simulink model "snap_fengine"  (R2016b)
settings: Solver=VariableStepDiscrete  StartTime=0.0  StopTime=10.0  RelTol=1e-3
libraries: xbsIndex_r4 x5026, casper_library_misc x38, xps_library x10, casper_library_delays x6, casper_library_sources x3, casper_library_reorder x2, casper_library_communications x1
(part 1 of 43)
settings Model: Creator=mdexter  LastModifiedBy=jackh
settings Model: ModifiedComment=|
  | jackh -- Sun Oct 27 09:17:26 2019 -- Version 1.368
  | compiled
settings Model: ModifiedHistory=|
  | jackh -- Sun Oct 27 09:17:26 2019 -- Version 1.368
  | compiled
  | 
  | jackh -- Sun Oct 27 07:24:12 2019 -- Version 1.367
  | remove registering of reorder outputs
  | 
  | jackh -- Sun Oct 27 07:22:37 2019 -- Version 1.366
  | change input snapshot to snap only one of 3 inputs
  | 
  | jackh -- Sun Oct 27 03:59:18 2019 -- Version 1.365
  | remove some superfluous registers to improve timing.
  | Reduce snapshot in input block from 1k samples to 512
  | 
  | jackh -- Sun Oct 27 01:46:50 2019 -- Version 1.364
  | Fix FFT shift bitwidth bug
  | 
  | FFT core was expecting a 16-bit shift, but only a 12bit value was sliced from the control register
  | 
  | jackh -- Fri Aug 30 09:22:01 2019 -- Version 1.363
  | compiled
  | 
  | jackh -- Thu Aug 29 17:13:27 2019 -- Version 1.362
  | change delay shift reg to 3 bit addr
  | 
  | jackh -- Thu Aug 29 11:33:13 2019 -- Version 1.361
  | corr fixes
  | 
  | jackh -- Thu Aug 29 11:09:21 2019 -- Version 1.360
  | latency fix in eqtvg
  | 
  | jackh -- Thu Aug 29 10:02:04 2019 -- Version 1.359
  | compiled
  | 
  | jackh -- Wed Aug 28 15:31:00 2019 -- Version 1.358
  | bump to version 1.3
  | 
  | jackh -- Wed Aug 28 15:26:18 2019 -- Version 1.357
  | change quantization to saturate.
  | Change coefficients to 16_5 (was 16_6)
  | 
  | jackh -- Wed Aug 28 14:17:28 2019 -- Version 1.356
  | remove debugging snapshots hidden in corr vaccs
  | 
  | jackh -- Fri Aug 23 15:01:55 2019 -- Version 1.355
  | compiled
  | 
  | jackh -- Fri Aug 23 10:43:05 2019 -- Version 1.354
  | add snapshot in input block
  | 
  | jackh -- Thu Aug 22 17:13:50 2019 -- Version 1.353
  | fix to eqtvg ram depths
  | 
  | jackh -- Thu Aug 22 15:23:14 2019 -- Version 1.352
  | bump version to 1.2
  | 
  | jackh -- Thu Aug 22 15:22:39 2019 -- Version 1.351
  | Force pairs of pols to have same random number generator to save resources
  | 
  | jackh -- Thu Aug 22 15:19:21 2019 -- Version 1.350
  | rotator channel index counter fixes
  | 
  | eq tvg split bram into 3 (so we can have 6 channels, not 8)
  | 
  | jackh -- Thu Aug 22 12:01:44 2019 -- Version 1.349
  | 
  | 
  | jackh -- Thu Aug 22 12:01:21 2019 -- Version 1.348
  | Changes to rotator precision
  | 
  | jackh -- Tue Aug 20 19:46:09 2019 -- Version 1.347
  | compiled
  | 
  | jackh -- Tue Aug 20 16:55:38 2019 -- Version 1.346
  | increase minimum walsh period to 2**18 fpga clocks (was 2**13)
  | 
  | jackh -- Tue Aug 20 16:40:34 2019 -- Version 1.345
  | 
  | 
  | jackh -- Tue Aug 20 16:15:18 2019 -- Version 1.344
  | bump version to 1.1
  | 
  | jackh -- Tue Aug 20 16:14:49 2019 -- Version 1.343
  | add global enables to phase switch mod/demod to make software easier
  | 
  | jackh -- Mon Aug 19 17:54:23 2019 -- Version 1.342
  | compiled
  | 
  | jackh -- Thu Aug 01 11:53:22 2019 -- Version 1.341
  | make programmable sync delay tolerate delay=0
  | 
  | jackh -- Wed Jul 31 13:49:54 2019 -- Version 1.340
  | comment out corr->rms
  | 
  | jackh -- Mon Jul 29 17:05:34 2019 -- Version 1.339
  | delete corr rms block (not currently enough ram)
  | 
  | jackh -- Mon Jul 29 17:03:29 2019 -- Version 1.338
  | Add version block
  | 
  | jackh -- Mon Jul 29 16:58:22 2019 -- Version 1.337
  | make sync in have a programmable delay
  | Solves 2 problems:
  | 
  | 1) Can start integrations at arbitrary times (good for LST alignment)
  | 2) Can start a 16 second integration chunk on an arbitrary time boundary (needed to avoid the downstream correlator having 16 second start / stop granularity)
  | 
  | jackh -- Mon Jul 29 16:50:03 2019 -- Version 1.336
  | update phasor to 24-bits
  | 
  | jackh -- Sat May 11 17:48:41 2019 -- Version 1.335
  | 
  | 
  | jackh -- Sat May 11 17:46:07 2019 -- Version 1.334
  | 
  | 
  | jackh -- Sat May 11 17:45:44 2019 -- Version 1.333
  | 
  | 
  | jackh -- Sat May 11 17:40:04 2019 -- Version 1.332
  | 
  | 
  | jackh -- Sat May 11 17:36:59 2019 -- Version 1.331
  | add vacc for autocorrs @ 16 bit resolution
  | 
  | deepthi -- Sun Oct 28 15:16:19 2018 -- Version 1.330
  | 
  | 
  | deepthi -- Sat Oct 27 18:45:54 2018 -- Version 1.329
  | 
  | packetizer: Added an 'and' block that holds new_packet signal in high until the first sync.
  | 
  | deepthi -- Sat Oct 27 17:33:32 2018 -- Version 1.328
  | 
  | 1. Change edge_detect location in sync block
  | 
  | deepthi -- Sat Oct 20 22:13:43 2018 -- Version 1.327
  | 
  | 1. Add edge detect to software reg and gpio input in sync block.
  | 
  | 2. Add new corr block with max hold functionality.
  | 
  | jackh -- Tue Oct 09 20:34:13 2018 -- Version 1.326
  | recompile with pmbus_alert register
  | 
  | jackh -- Thu Jul 12 10:55:28 2018 -- Version 1.325
  | 
  | 
  | jackh -- Wed Jul 11 17:20:51 2018 -- Version 1.324
  | syntax
  | 
  | jackh -- Wed Jul 11 17:16:24 2018 -- Version 1.323
  | increase resolution of phase rotator bram.
  | 
  | jackh -- Wed Jul 11 17:10:41 2018 -- Version 1.322
  | 
  | 
  | jackh -- Tue Jul 10 16:08:30 2018 -- Version 1.321
  | scramble rotator channel multiplers to match PFB output order (hopefully)
  | 
  | jackh -- Tue Jul 10 15:51:56 2018 -- Version 1.320
  | 
  | 
  | jackh -- Tue Jul 10 13:37:24 2018 -- Version 1.319
  | fix off-by-one in slicing of mcnt counter, which was having the effect of duplicating mcnts in headers
  | 
  | jackh -- Sat Jul 07 14:17:05 2018 -- Version 1.318
  | compiled
  | 
  | jackh -- Fri Jul 06 10:33:47 2018 -- Version 1.317
  | fix bitbashing to rotator phase addresses
  | 
  | jackh -- Fri Jul 06 10:17:15 2018 -- Version 1.316
  | Add mux to enable / disable rotator
  | 
  | jackh -- Thu Jul 05 17:21:10 2018 -- Version 1.315
  | make some delays behavioural
  | 
  | jackh -- Thu Jul 05 14:48:28 2018 -- Version 1.314
  | 
  | 
  | jackh -- Thu Jul 05 14:46:13 2018 -- Version 1.313
  | 
  | 
  | jackh -- Thu Jul 05 14:43:36 2018 -- Version 1.312
  | 
  | 
  | jackh -- Thu Jul 05 14:40:00 2018 -- Version 1.311
  | 
  | 
  | jackh -- Thu Jul 05 14:36:19 2018 -- Version 1.310
  | 
  | 
  | jackh -- Thu Jul 05 14:26:16 2018 -- Version 1.309
  | integrate rotator into pipeline
  | 
  | jackh -- Thu Jul 05 14:20:20 2018 -- Version 1.308
  | 
  | create phase-rotation block
  | 
  | deepthi -- Thu Jun 07 09:24:03 2018 -- Version 1.307
  | 
  | Replaced the corr block.
  | 
  | deepthi -- Wed Jun 06 12:07:26 2018 -- Version 1.306
  | 
  | 
  | deepthi -- Tue Jun 05 17:46:17 2018 -- Version 1.305
  | 
  | Replaced the corr block with the tested version
  | 
  | deepthi -- Sat May 12 19:11:02 2018 -- Version 1.304
  | 
  | Changed time counter to increment between even/odd banks
  | 
  | deepthi -- Sat May 12 19:06:34 2018 -- Version 1.303
  | 
  | changed timing of eof, valid, data and headers
  | 
  | deepthi -- Mon May 07 23:03:07 2018 -- Version 1.302
  | 
  | 
  | deepthi -- Mon May 07 00:31:44 2018 -- Version 1.301
  | 
  | 
  | deepthi -- Fri May 04 20:13:43 2018 -- Version 1.300
  | 
  | Reduced width sliced from time_ctr
  | 
  | deepthi -- Fri May 04 19:47:57 2018 -- Version 1.299
  | 
  | Added delay to header and ip signals to account for pulse_ext on valid.
  | 
  | deepthi -- Fri May 04 19:23:23 2018 -- Version 1.298
  | 
  | 
  | deepthi -- Thu May 03 16:58:39 2018 -- Version 1.297
  | 
  | 1. Added delays to eof and dest_ip  to account for pulse_ext in valid.
  | 
  | 2. Changed eth_sw expected packet length to include header.
  | 
  | jackh -- Tue May 01 20:38:09 2018 -- Version 1.296
  | compiled
  | 
  | jackh -- Tue May 01 17:49:38 2018 -- Version 1.295
  | Fix to packetizer valid generation, to take into account the 3 (one per antenna) blocks of valid data in each stream of 512 channels
  | 
  | jackh -- Tue May 01 16:49:02 2018 -- Version 1.294
  | make channel selection bram 32-bits wide.
  | 
  | Remove GPU-packing mux / swreg
  | 
  | jackh -- Tue May 01 14:24:16 2018 -- Version 1.293
  | 
  | 
  | jackh -- Tue May 01 14:20:01 2018 -- Version 1.292
  | update chan reorderer
  | 
  | jackh -- Tue May 01 11:43:41 2018 -- Version 1.291
  | compiled
  | 
  | jackh -- Tue May 01 09:44:03 2018 -- Version 1.290
  | 
  | 
  | jackh -- Tue May 01 09:43:34 2018 -- Version 1.289
  | use bram for eq fft descramble map
  | 
  | jackh -- Tue May 01 09:40:26 2018 -- Version 1.288
  | change architecture of corr block -- now stores desired antennas in bram, rather than using a delay tree
  | 
  | jackh -- Mon Apr 30 20:21:35 2018 -- Version 1.287
  | 
  | 
  | jackh -- Mon Apr 30 20:18:20 2018 -- Version 1.286
  | 
  | 
  | jackh -- Mon Apr 30 20:15:51 2018 -- Version 1.285
  | compensate for FFT scrambling in EQ block. Descramble FFT post-requantization in this block
  | 
  | jackh -- Mon Apr 30 19:27:42 2018 -- Version 1.284
  | plausibility pass on corr block
  | 
  | jackh -- Mon Apr 30 12:16:47 2018 -- Version 1.283
  | 
  | 
  | jackh -- Mon Apr 30 12:14:25 2018 -- Version 1.282
  | store chan_reorder reorder map in bram
  | 
  | jackh -- Mon Apr 30 12:05:02 2018 -- Version 1.281
  | remove per-antenna histograms -- now get one histogram with multiplexed input
  | 
  | jackh -- Sun Apr 29 15:50:16 2018 -- Version 1.280
  | 
  | 
  | jackh -- Sun Apr 29 15:37:38 2018 -- Version 1.279
  | 
  | 
  | jackh -- Sun Apr 29 15:27:38 2018 -- Version 1.278
  | First pass packetizer. Regenerate pfb with parameter for serial block inputs
  | 
  | jackh -- Sat Mar 03 12:52:57 2018 -- Version 1.277
  | 
  | 
  | jackh -- Sun Feb 25 12:27:48 2018 -- Version 1.276
  | add pre-pfb reorder
  | 
  | jackh -- Sat Feb 24 13:39:06 2018 -- Version 1.275
  | 
  | jackh -- Sat Feb 24 13:38:40 2018 -- Version 1.274
  | update pfb to 16 inputs
  | 
  | jackh -- Fri Feb 23 18:44:26 2018 -- Version 1.273
  | 
  | 
  | jackh -- Fri Feb 23 18:38:20 2018 -- Version 1.272
  | 
  | 
  | jackh -- Fri Feb 23 17:01:30 2018 -- Version 1.271
  | make fft 8 parallel input
  | 
  | jackh -- Sat Feb 10 13:53:12 2018 -- Version 1.270
  | 
  | 
  | jackh -- Sat Feb 10 13:50:10 2018 -- Version 1.269
  | 
  | 
  | jackh -- Sat Feb 10 13:48:56 2018 -- Version 1.268
  | remove fft preshift
  | 
  | jackh -- Sat Feb 10 13:47:39 2018 -- Version 1.267
  | 
  | 
  | jackh -- Sat Feb 10 13:44:29 2018 -- Version 1.266
  | 
  | 
  | jackh -- Sat Feb 10 13:43:22 2018 -- Version 1.265
  | make delayer dual-pol
  | 
  | jackh -- Sat Feb 10 13:40:59 2018 -- Version 1.264
  | first pass new packet format with no time-based corner turn
  | 
  | jackh -- Fri Feb 09 17:29:05 2018 -- Version 1.263
  | 
  | 
  | jackh -- Fri Feb 09 15:23:03 2018 -- Version 1.262
  | first pass turning everything to 8192 channels
  | 
  | Changed the ants addr to be driven by the same signal that drives chans, ips (used to be driven by ant_tracker).
  | 
  | Removed nants software register that was previously thought to control time stamps (but didn't really)
  | 
  | deepthi -- Wed Jan 31 18:20:45 2018 -- Version 1.261
  | 
  | deepthi -- Mon Jan 29 17:20:36 2018 -- Version 1.260
  | 
  | 
  | deepthi -- Mon Jan 29 17:18:54 2018 -- Version 1.259
  | 
  | 
  | deepthi -- Mon Jan 29 17:18:33 2018 -- Version 1.258
  | 
  | 
  | deepthi -- Mon Jan 29 16:51:19 2018 -- Version 1.257
  | 
  | 
  | deepthi -- Mon Jan 29 16:46:46 2018 -- Version 1.256
  | 
  | 
  | deepthi -- Mon Jan 29 16:37:32 2018 -- Version 1.255
  | 
  | 
  | deepthi -- Mon Jan 29 16:11:03 2018 -- Version 1.254
  | 
  | 
  | deepthi -- Mon Jan 29 15:55:33 2018 -- Version 1.253
  | 
  | 
  | jackh -- Fri Nov 17 19:04:05 2017 -- Version 1.252
  | compiled
  | 
  | jackh -- Wed Nov 15 11:31:03 2017 -- Version 1.251
  | go to 3 corr blocks
  | 
  | jackh -- Tue Nov 14 16:10:40 2017 -- Version 1.250
  | 
  | 
  | jackh -- Tue Nov 14 15:28:37 2017 -- Version 1.249
  | reduce bram use in histogram shared brams
  | 
  | jackh -- Mon Nov 13 18:55:18 2017 -- Version 1.248
  | fix bug in histogram shared bram addr width
  | 
  | jackh -- Fri Nov 10 17:05:56 2017 -- Version 1.247
  | add 4 independent corr subsystems. Add EQ clipping counters
  | 
  | jackh -- Fri Nov 10 14:21:14 2017 -- Version 1.246
  | 
  | 
  | jackh -- Fri Nov 10 14:19:27 2017 -- Version 1.245
  | 
  | 
  | jackh -- Fri Nov 10 11:40:47 2017 -- Version 1.244
  | update to histograms v2
  | 
  | jackh -- Tue Nov 07 22:23:59 2017 -- Version 1.243
  | compiled -- passes eqtvg
  | 
  | jackh -- Tue Nov 07 20:41:00 2017 -- Version 1.242
  | 
  | 
  | jackh -- Tue Nov 07 20:39:30 2017 -- Version 1.241
  | packet header generation fixes
  | 
  | jackh -- Tue Nov 07 17:19:53 2017 -- Version 1.240
  | 
  | 
  | jackh -- Tue Nov 07 17:14:47 2017 -- Version 1.239
  | 
  | 
  | jackh -- Tue Nov 07 17:08:29 2017 -- Version 1.238
  | remove some chan_reorder debug snapshots
  | 
  | jackh -- Tue Nov 07 17:06:39 2017 -- Version 1.237
  | update ps GPIO pins
  | 
  | **** Change packetizer header blocks to can have a separate antenna / ip / chan for each packet. This is for the nants > 3 simulation modes. This will break previous versions of software *****
  | 
  | jackh -- Mon Nov 06 22:06:03 2017 -- Version 1.236
  | add comment to corr_acc_len
  | 
  | Compiled -- passes EQTVG test!
  | 
  | jackh -- Mon Nov 06 15:24:31 2017 -- Version 1.235
  | add OR block in mrst generator so that counter is enabled if/when an arm signal comes
  | 
  | jackh -- Sun Nov 05 21:39:25 2017 -- Version 1.234
  | comment on sync period
  | 
  | jackh -- Sun Nov 05 17:39:01 2017 -- Version 1.233
  | fix bitbasher in 32-spectra corner turn
  | 
  | jackh -- Sun Nov 05 17:05:17 2017 -- Version 1.232
  | aesthetic
  | 
  | jackh -- Sun Nov 05 17:02:53 2017 -- Version 1.231
  | changes to comments
  | 
  | jackh -- Sun Nov 05 17:01:27 2017 -- Version 1.230
  | make acc_len it's own register so we can acc to 2**32
  | 
  | jackh -- Sun Nov 05 16:58:57 2017 -- Version 1.229
  | 
  | 
  | jackh -- Sun Nov 05 16:56:52 2017 -- Version 1.228
  | add internal correlator
  | 
  | jackh -- Sun Nov 05 16:24:21 2017 -- Version 1.227
  | compiled.
  | 
  | jackh -- Sun Nov 05 15:19:13 2017 -- Version 1.226
  | latency tweak to data line in packetizer
  | 
  | jackh -- Sat Nov 04 20:21:54 2017 -- Version 1.225
  | change ethernet debug counters to 32 bits
  | 
  | jackh -- Sat Nov 04 20:05:10 2017 -- Version 1.224
  | make chan reorder map bram 32 bits to aid with software
  | 
  | jackh -- Sat Nov 04 19:51:25 2017 -- Version 1.223
  | change header brams to be 32-bit wide for all values.
  | This makes it easier to deal with the software, which can only write 32-bit bounded words.
  | 
  | jackh -- Sat Nov 04 14:23:39 2017 -- Version 1.222
  | replace big distributed ram in 16-spectra corner turn
  | with simple bit basher manipulation. The distributed ram tool a ridiculous amount of time to synthesize. Hopefully this will be faster.
  | 
  | jackh -- Fri Nov 03 16:25:40 2017 -- Version 1.221
  | 
  | 
  | jackh -- Fri Nov 03 16:17:13 2017 -- Version 1.220
  | update casper blocks on phase switch subsys
  | 
  | jackh -- Fri Nov 03 16:14:34 2017 -- Version 1.219
  | 
  | 
  | jackh -- Fri Nov 03 13:09:23 2017 -- Version 1.218
  | add phase switching and i2c control
  | 
  | jackh -- Fri Nov 03 12:43:29 2017 -- Version 1.217
  | 
  | add i2C controllers
  | 
  | jackh -- Mon Oct 23 16:15:14 2017 -- Version 1.216
  | Add back in Deepthi's fix from f3b63dae07d62
  | 
  | jackh -- Mon Oct 23 16:04:59 2017 -- Version 1.215
  | 
  | 
  | jackh -- Mon Oct 23 14:44:02 2017 -- Version 1.214
  | compiled. Still minor timing errors in the histograms
  | 
  | jackh -- Mon Oct 23 10:40:37 2017 -- Version 1.213
  | change EQ coeffs to one-per channel. Make format 16_6 (was 18_7)
  | 
  | jackh -- Mon Oct 09 15:00:17 2017 -- Version 1.212
  | 
  | halve number of brams in histogram readout
  | 
  | jackh -- Wed Sep 13 11:46:17 2017 -- Version 1.211
  | use built-in tge status regs
  | 
  | jackh -- Tue Sep 12 21:14:25 2017 -- Version 1.210
  | 
  | 
  | jackh -- Tue Sep 12 21:10:57 2017 -- Version 1.209
  | update_casper_blocks(bdroot)
  | 
  | jackh -- Tue Sep 12 21:02:11 2017 -- Version 1.208
  | add histogram to adc stats
  | 
  | jackh -- Fri Jul 14 11:30:38 2017 -- Version 1.207
  | set map = reord_map in chan_reorder blocks which use matlab scripts to generate their reorders.
  | 
  | jackh -- Thu Jul 13 17:48:05 2017 -- Version 1.206
  | change sync period to a 32-bit sw reg (was hardcoded 9! * 1024)
  | 
  | deepthi -- Thu Jul 13 13:07:36 2017 -- Version 1.205
  | 
  | 
  | deepthi -- Thu Jul 13 12:10:35 2017 -- Version 1.204
  | 
  | 
  | deepthi -- Wed Jul 12 16:52:46 2017 -- Version 1.203
  | 
  | 
  | deepthi -- Wed Jul 12 15:57:48 2017 -- Version 1.202
  | 
  | 
  | deepthi -- Tue Jul 11 19:00:41 2017 -- Version 1.201
  | 
  | 
  | deepthi -- Tue Jul 11 18:54:05 2017 -- Version 1.200
  | 
  | 
  | deepthi -- Tue Jul 11 18:52:32 2017 -- Version 1.199
  | 
  | 
  | deepthi -- Mon Jul 10 16:18:51 2017 -- Version 1.198
  | 
  | 
  | deepthi -- Sun Jul 09 18:15:02 2017 -- Version 1.197
  | 
  | 
  | deepthi -- Thu Jul 06 13:54:16 2017 -- Version 1.196
  | 
  | 
  | jackh -- Mon Jul 03 11:01:40 2017 -- Version 1.195
  | 
  | 
  | jackh -- Fri Jun 30 13:59:17 2017 -- Version 1.194
  | enable CPU tx/rx buffer on tge core. Needed for microblaze.
  | 
  | jackh -- Mon Jun 26 11:33:24 2017 -- Version 1.193
  | 
  | 
  | jackh -- Thu Jun 22 14:37:16 2017 -- Version 1.192
  | add history prompting
settings DataIOCC: LimitDataPoints=on  SaveFormat=Array  SignalLoggingSaveFormat=ModelDataLogs
settings OptimizationCC: DefaultParameterBehavior=Inlined  ExpressionDepthLimit=2147483647  LifeSpan=inf
settings DebuggingCC: UnderspecifiedInitializationDetection=Classic  MergeDetectMultiDrivingBlocksExec=none  SolverPrmCheckMsg=warning  FcnCallInpInsideContextMsg=warning  AllowSymbolicDim=off  StateNameClashWarn=warning  SFUnexpectedBacktrackingDiag=warning  SFNoUnconditionalDefaultTransitionDiag=warning  SFExecutionAtInitializationDiag=none
settings HardwareCC: ProdBitPerPointer=32  ProdBitPerSizeT=32  ProdBitPerPtrDiffT=32  ProdLargestAtomicFloat=None  ProdIntDivRoundTo=Undefined  ProdEndianess=Unspecified  ProdWordSize=32  ProdHWDeviceType=32-bit Generic
settings ModelReferenceCC: PropagateSignalLabelsOutOfModel=off
settings GRTTargetCC: TargetLangStandard=C89/C90 (ANSI)  GeneratePreprocessorConditionals=Disable all  CombineOutputUpdateFcns=off  GRTInterface=on
settings ConfigComp: CovMetricSettings=dw  CovHtmlReporting=on  CovSaveCumulativeToWorkspaceVar=on  CovSaveSingleToWorkspaceVar=on  CovExternalEMLEnable=off

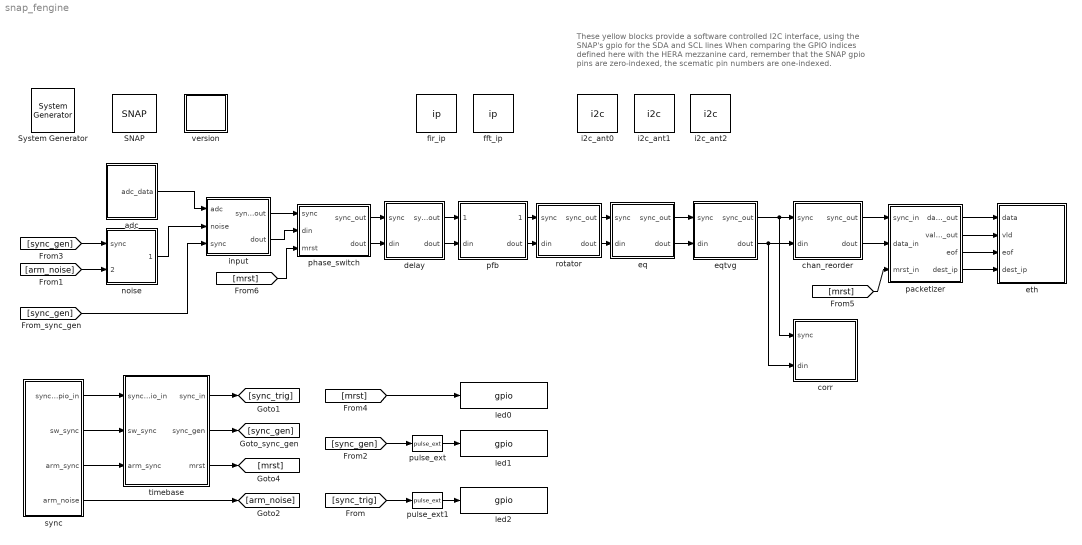
== system snap_fengine ==
  note: These yellow blocks provide a software controlled I2C interface, using
      | the SNAP's gpio for the SDA and SCL lines
      | When comparing the GPIO indices defined here with the HERA
      | mezzanine card, remember that the SNAP gpio pins are zero-indexed,
      | the scematic pin numbers are one-indexed.
  " System Generator" : xbsIndex_r4/ System Generator  Tag=genX  xilinxfamily=kintex7  part=xc7k160t  speed=-2  package=ffg676  synthesis_tool=XST  clock_wrapper=Clock Enables  directory=/data/home/jackh/herafengine/snap_fengine/sysgen  proj_type=Vivado  Synth_file=Vivado Synthesis Defaults  Impl_file=Vivado Implementation Defaults  testbench=off  simulink_period=1  sysclk_period=4  dcm_input_clock_period=10  incr_netlist=off  trim_vbits=Everywhere in SubSystem  dbl_ovrd=According to Block Masks  core_generation=According to Block Masks  run_coregen=off  deprecated_control=off  eval_field=0  block_type=sysgen
  SNAP : xps_library/Platforms/SNAP  Tag=xps:xsg  hw_sys=SNAP:xc7k160t  clk_src=adc0_clk  clk_rate=250  use_microblaze=on  sample_period=1  synthesis_tool=XST
  adc : Subsystem
  chan_reorder : Subsystem
  corr : Subsystem
  delay : Subsystem
  eq : Subsystem
  eqtvg : Subsystem
  eth : Subsystem
  fft_ip : xps_library/ip  Tag=xps:ip  lib_path=[fileparts(which(gcs)) '/fft_8192_1a_core']  ip_name='fft_8192_1a_core'
  fir_ip : xps_library/ip  Tag=xps:ip  lib_path=[fileparts(which(gcs)) '/pfb_fir_8192ch_core']  ip_name='pfb_fir_8192ch_core'
  i2c_ant0 : xps_library/i2c  Tag=xps:i2c  sda_gpio='rpi_header'  sda_gpio_index=6  scl_gpio='rpi_header'  scl_gpio_index=7
  i2c_ant1 : xps_library/i2c  Tag=xps:i2c  sda_gpio='rpi_header'  sda_gpio_index=30  scl_gpio='rpi_header'  scl_gpio_index=31
  i2c_ant2 : xps_library/i2c  Tag=xps:i2c  sda_gpio='rpi_header'  sda_gpio_index=35  scl_gpio='rpi_header'  scl_gpio_index=36
  input : Subsystem
  led0 : xps_library/gpio  Tag=xps:gpio  io_group=ROACH2:led  io_group_custom=0  io_dir=out  arith_type=Boolean  bitwidth=1  bin_pt=0  bit_index=0  sample_period=1  use_single_ended=off  use_ddr=off  reg_iob=on  reg_clk_phase=0  termination=None
  led1 : xps_library/gpio  Tag=xps:gpio  io_group=ROACH2:led  io_group_custom=0  io_dir=out  arith_type=Boolean  bitwidth=1  bin_pt=0  bit_index=1  sample_period=1  use_single_ended=off  use_ddr=off  reg_iob=on  reg_clk_phase=0  termination=None
  led2 : xps_library/gpio  Tag=xps:gpio  io_group=ROACH2:led  io_group_custom=0  io_dir=out  arith_type=Boolean  bitwidth=1  bin_pt=0  bit_index=2  sample_period=1  use_single_ended=off  use_ddr=off  reg_iob=on  reg_clk_phase=0  termination=None
  noise : Subsystem
  packetizer : Subsystem  mask{nchan_bits=13, nsamp_per_pkt=2, nchan_per_pkt=384, nant_per_pkt=3, nants=4, clks_per_pkt=512/8*4*2*2, pkts_per_cycle=16*2, chan_frac_sent=384/512}
      mask prompts: nchan_bits "Number of channels (including unsent) (2^?)"; nsamp_per_pkt "Time samples per packet"; nchan_per_pkt "Channels per packet"; nant_per_pkt "Antennas per packet"; nants "Number of antennas including dummys"; clks_per_pkt "Send packet every ? clocks"; pkts_per_cycle "Packets per cycle"; chan_frac_sent "Fraction of channels sent"
      mask init:
      | nwords = nchan_per_pkt * nsamp_per_pkt * nant_per_pkt * 2 / 8
      | 
      | % +1 for dual-pol => 2 bytes per sample
      | % -3 for 2^3 = 8 bytes per word
      | 
      | clks_to_eof = (512*nsamp_per_pkt*nant_per_pkt*2/8) -(512*nsamp_per_pkt*2)/(4*8)
      | 
      | % 512 (including channels not sent)
      | % -512/4. to account for (1-chan_frac_sent) valid=0
  pfb : Subsystem
  phase_switch : Subsystem
  pulse_ext : casper_library_misc/pulse_ext  pulse_len=2^26
  pulse_ext1 : casper_library_misc/pulse_ext  pulse_len=2^26
  rotator : Subsystem  mask{chan_bits=13, pchan_bits=3, npol_bits=3, spectra_share_bits=10, spectra_bits=19}
      mask prompts: chan_bits "Number of channels (2^?)"; pchan_bits "Parallel channels (2^?)"; npol_bits "Number of polarizations (2^?) (Sequential polarization pairs are assumed to be from the same antenna, and get the same phase)"; spectra_share_bits "Increment phase every how many spectra (2^?)"; spectra_bits "Maximum number of spectra to phase (2^?)"
  sync : Subsystem
  timebase : Subsystem
  version : Subsystem  mask{ver_maj=1, ver_min=4}
      mask prompts: ver_maj "Major version"; ver_min "Minor version"
  wires:
  adc/1(adc_data) -> input/1(adc)
  noise/1(noise) -> input/2(noise)
  sync/1(sync_gpio_in) -> timebase/1(sync_gpio_in)
  sync/2(sw_sync) -> timebase/2(sw_sync)
  sync/3(arm_sync) -> timebase/3(arm_sync)
  [arm_noise] -> noise/2(arm_ld)
  [sync_gen] -> noise/1(sync)
  timebase/2(sync_gen) -> [sync_gen]
  timebase/1(sync_in) -> [sync_trig]
  sync/4(arm_noise) -> [arm_noise]
  [sync_gen] -> input/3(sync)
  eq/1(sync_out) -> eqtvg/1(sync)
  eq/2(dout) -> eqtvg/2(din)
  eqtvg/1(sync_out) -> corr/1(sync), chan_reorder/1(sync)
  eqtvg/2(dout) -> corr/2(din), chan_reorder/2(din)
  packetizer/1(data_out) -> eth/1(data)
  packetizer/2(valid_out) -> eth/2(vld)
  packetizer/3(eof) -> eth/3(eof)
  packetizer/4(dest_ip) -> eth/4(dest_ip)
  timebase/3(mrst) -> [mrst]
  [sync_gen] -> pulse_ext/1
  [mrst] -> led0/1
  pulse_ext/1 -> led1/1
  delay/1(sync_out) -> pfb/1(sync_in)
  delay/2(dout) -> pfb/2(din)
  [sync_trig] -> pulse_ext1/1
  pulse_ext1/1 -> led2/1
  input/1(sync_out) -> phase_switch/1(sync)
  phase_switch/2(dout) -> delay/2(din)
  phase_switch/1(sync_out) -> delay/1(sync)
  input/2(dout) -> phase_switch/2(din)
  [mrst] -> phase_switch/3(mrst)
  chan_reorder/1(sync_out) -> packetizer/1(sync_in)
  chan_reorder/2(dout) -> packetizer/2(data_in)
  [mrst] -> packetizer/3(mrst_in)
  pfb/1(sync_out) -> rotator/1(sync)
  pfb/2(dout) -> rotator/2(din)
  rotator/1(sync_out) -> eq/1(sync)
  rotator/2(dout) -> eq/2(din)

== system snap_fengine/adc ==
  Assert{,1..11} (12 alike) : xbsIndex_r4/Assert  assert_type=off  type_source=Explicitly  gui_display_data_type=Fixed-point  arith_type="Signed  (2's comp)"  n_bits=16  bin_pt=14  preci_type=Single  exp_width=8  frac_width=24  assert_rate=on  rate_source=Explicitly  period=1  output_port=on  block_type=assert
  Constant{4..13,33..34} (12 alike) : Constant  Value=0
  bus_create : Subsystem  AncestorBlock=casper_library_flow_control/bus_create  mask(bus_create){inputNum=12}
      mask prompts: inputNum "Number of inputs:"
      mask init:
      | bus_create_init(gcb,...
      |     'inputNum', inputNum);
  snap_adc : Subsystem  Tag=xps:snap_adc  AncestorBlock=xps_library/ADCs/snap_adc  mask(adc_snap){sample_rate=500, snap_inputs=6, adc_resolution=8}
      mask prompts: sample_rate "Sample rate (MHz)"; snap_inputs "Number of inputs per snap"; adc_resolution "Resolution of ADC (number of bit)"
      mask help: Interface to the 3 adc chips on the SNAP board. Please see Help for instructions on parameter settings
      mask init:
      | adc_snap_init(gcb);
      mask Help:
      | This is the CASPER "yellow block" for the ADCs on the SNAP board.
      | Each ADC chip accepts four inputs.
      | 
      | Maximum sample rate f (Mega samples per second)
      | 
      | Number of inputs         3                6                12
      | Resolution 8 bits          f=1000      f=500         f=250
      | Resolution 12 bits        f=640        f=320         f=160
      | 
      | Resolution 12 bits is available when SNAP board is upgraded with HMCAD1520 ADC chips
      mask TypeOptions snap_inputs: 3 | 6 | 12
      mask TypeOptions adc_resolution: 8 | 12
  adc_data : Outport
  wires:
  Constant4/1 -> snap_adc/1(a1_sim)
  Constant5/1 -> snap_adc/2(a2_sim)
  Constant6/1 -> snap_adc/3(a3_sim)
  Constant7/1 -> snap_adc/4(a4_sim)
  Constant8/1 -> snap_adc/5(b1_sim)
  Constant9/1 -> snap_adc/6(b2_sim)
  Constant33/1 -> snap_adc/7(b3_sim)
  Constant34/1 -> snap_adc/8(b4_sim)
  Constant10/1 -> snap_adc/9(c1_sim)
  Constant11/1 -> snap_adc/10(c2_sim)
  Constant12/1 -> snap_adc/11(c3_sim)
  Constant13/1 -> snap_adc/12(c4_sim)
  bus_create/1(bus_out) -> adc_data/1
  snap_adc/1(a1) -> Assert/1  "in0"
  snap_adc/2(a2) -> Assert1/1  "in1"
  snap_adc/3(a3) -> Assert2/1  "in2"
  snap_adc/4(a4) -> Assert3/1  "in3"
  snap_adc/5(b1) -> Assert4/1  "in4"
  snap_adc/6(b2) -> Assert5/1  "b2"
  snap_adc/7(b3) -> Assert6/1  "b3"
  snap_adc/8(b4) -> Assert7/1  "b4"
  snap_adc/9(c1) -> Assert8/1  "c1"
  snap_adc/10(c2) -> Assert9/1  "c2"
  snap_adc/11(c3) -> Assert10/1  "c3"
  snap_adc/12(c4) -> Assert11/1  "c4"
  Assert/1 -> bus_create/1(in1)
  Assert1/1 -> bus_create/2(in2)
  Assert2/1 -> bus_create/3(in3)
  Assert3/1 -> bus_create/4(in4)
  Assert6/1 -> bus_create/7(in7)
  Assert7/1 -> bus_create/8(in8)
  Assert5/1 -> bus_create/6(in6)
  Assert4/1 -> bus_create/5(in5)
  Assert9/1 -> bus_create/10(in10)
  Assert8/1 -> bus_create/9(in9)
  Assert11/1 -> bus_create/12(in12)
  Assert10/1 -> bus_create/11(in11)

== system snap_fengine/chan_reorder ==
  note: Mess with the parallel ordering so that channels don't increment
      | by 8 at every step
  note: Use this programmable
      | map to mess with the channel
      | ordering.
      |
      | Out of every block of 512 channels,
      | only the first 384 will be sent.
      | So fold the edges of the band into unwanted slots
  note: Go from an array ordered Nt*Na*Np*Nb*Nc (times[2] x antennas[4] x pols[2] x blocks-per-spectra[16] x channels-per-block[64])
      | to one ordered:
      | Nb*Na*Nc*Nt*Np
      |
      | reshape(permute(reshape(x, Nc, Nb, Np, Na, Nt), [3 5 1 4 2]), Nb*Na*Nc*Nt*Np, 1)
      |
      | i.e. reshape(permute(reshape([0 : 2*4*2*16*64 - 1], 64, 16, 2, 4, 2), [3 5 1 4 2]), 2*4*2*16*64, 1)
  note: input order is:
      | a0, a8, ... a8184, b0, b8, ..., b8184, ..., f0, f8, ..., f8184, X0, X8, ..., X8184
      | ...
      | a7, a15, ... a8191, b7, b15, ..., b8191, ..., f7, f15, ..., f8191, X7, X15, ..., X8191
      |
      | (i.e., a single 8192 channel spectra, 8 channels at a time, for 6 real polarizations (a through f),
      | and two dummy polarizations).
      | A complete cycle takes 8192 (channels) / 8 (channels in parallel) * 8 (pols including dummys) = 8192 clocks
  sync : Inport
  din : Inport  Port=2
  Constant : xbsIndex_r4/Constant  const=1  gui_display_data_type=Boolean  arith_type=Boolean  n_bits=1  bin_pt=0  preci_type=Single  exp_width=8  frac_width=24  explicit_period=on  period=1  equ=P=C  opselect=C  inp2=PCIN>>17  opr=+  inp1=P  carry=CIN  dbl_ovrd=off  block_type=constant
  Constant1 : xbsIndex_r4/Constant  const=1  gui_display_data_type=Boolean  arith_type=Boolean  n_bits=1  bin_pt=0  preci_type=Single  exp_width=8  frac_width=24  explicit_period=on  period=1  equ=P=C  opselect=C  inp2=PCIN>>17  opr=+  inp1=P  carry=CIN  dbl_ovrd=off  block_type=constant
  Constant2 : xbsIndex_r4/Constant  const=1  gui_display_data_type=Boolean  arith_type=Boolean  n_bits=1  bin_pt=0  preci_type=Single  exp_width=8  frac_width=24  explicit_period=on  period=1  equ=P=C  opselect=C  inp2=PCIN>>17  opr=+  inp1=P  carry=CIN  dbl_ovrd=off  block_type=constant
  bus_create : Subsystem  AncestorBlock=casper_library_flow_control/bus_create  mask(bus_create){inputNum=4}
      mask prompts: inputNum "Number of inputs:"
      mask init:
      | bus_create_init(gcb,...
      |     'inputNum', inputNum);
  bus_create1 : Subsystem  AncestorBlock=casper_library_flow_control/bus_create  mask(bus_create){inputNum=4}
      mask prompts: inputNum "Number of inputs:"
      mask init:
      | bus_create_init(gcb,...
      |     'inputNum', inputNum);
  bus_create2 : Subsystem  AncestorBlock=casper_library_flow_control/bus_create  mask(bus_create){inputNum=2}
      mask prompts: inputNum "Number of inputs:"
      mask init:
      | bus_create_init(gcb,...
      |     'inputNum', inputNum);
  bus_expand : Subsystem  AncestorBlock=casper_library_flow_control/bus_expand  mask(bus_expand){mode=divisions of equal size, outputNum=4, outputWidth=8, outputBinaryPt=0, outputArithmeticType=0, show_format=off, outputToWorkspace=off, variablePrefix=out, outputToModelAsWell=on}
      mask prompts: outputNum "Number of outputs:"; outputWidth "Output width:"; outputBinaryPt "Output binary point position:"; outputArithmeticType "Output arithmetic type (ufix=0, fix=1, bool=2):"; show_format "Print format string?"; outputToWorkspace "Output to workspace?"; variablePrefix "Variable name prefix:"; outputToModelAsWell "Output to model as well?"
      mask help:
      | Expands a 'bus' made using a bus_create or Xilinx
      | concat block.
      | The input will be divided into the specified number
      | of outputs with the specified arithmetic types.
      | Divisions are made from most significant bit.
      mask init:
      | bus_expand_init(gcb,...
      |     'mode', mode, ...
      |     'outputNum', outputNum, ...
      |     'outputWidth', outputWidth, ...
      |     'outputBinaryPt', outputBinaryPt, ...
      |     'outputArithmeticType', outputArithmeticType, ...
      |     'show_format', show_format, ...
      |     'outputToWorkspace', outputToWorkspace, ...
      |     'variablePrefix', variablePrefix, ...
      |     'outputToModelAsWell', outputToModelAsWell);
      settings: AttributesFormatString=4 outputs
      mask TypeOptions mode: divisions of equal size | divisions of arbitrary size
      mask Callback mode: bus_expand_callback();
      mask Callback outputWidth: bus_expand_callback();
      mask Callback outputToWorkspace: bus_expand_callback();
  bus_expand1 : Subsystem  AncestorBlock=casper_library_flow_control/bus_expand  mask(bus_expand){mode=divisions of equal size, outputNum=2, outputWidth=32, outputBinaryPt=0, outputArithmeticType=0, show_format=off, outputToWorkspace=off, variablePrefix=out, outputToModelAsWell=on}
      mask prompts: outputNum "Number of outputs:"; outputWidth "Output width:"; outputBinaryPt "Output binary point position:"; outputArithmeticType "Output arithmetic type (ufix=0, fix=1, bool=2):"; show_format "Print format string?"; outputToWorkspace "Output to workspace?"; variablePrefix "Variable name prefix:"; outputToModelAsWell "Output to model as well?"
      mask help:
      | Expands a 'bus' made using a bus_create or Xilinx
      | concat block.
      | The input will be divided into the specified number
      | of outputs with the specified arithmetic types.
      | Divisions are made from most significant bit.
      mask init: same as snap_fengine/chan_reorder/bus_expand
      settings: AttributesFormatString=2 outputs
      mask TypeOptions mode: divisions of equal size | divisions of arbitrary size
      mask Callback mode: bus_expand_callback();
      mask Callback outputWidth: bus_expand_callback();
      mask Callback outputToWorkspace: bus_expand_callback();
  bus_expand2 : Subsystem  AncestorBlock=casper_library_flow_control/bus_expand  mask(bus_expand){mode=divisions of equal size, outputNum=4, outputWidth=8, outputBinaryPt=0, outputArithmeticType=0, show_format=off, outputToWorkspace=off, variablePrefix=out, outputToModelAsWell=on}
      mask prompts: outputNum "Number of outputs:"; outputWidth "Output width:"; outputBinaryPt "Output binary point position:"; outputArithmeticType "Output arithmetic type (ufix=0, fix=1, bool=2):"; show_format "Print format string?"; outputToWorkspace "Output to workspace?"; variablePrefix "Variable name prefix:"; outputToModelAsWell "Output to model as well?"
      mask help:
      | Expands a 'bus' made using a bus_create or Xilinx
      | concat block.
      | The input will be divided into the specified number
      | of outputs with the specified arithmetic types.
      | Divisions are made from most significant bit.
      mask init: same as snap_fengine/chan_reorder/bus_expand
      settings: AttributesFormatString=4 outputs
      mask TypeOptions mode: divisions of equal size | divisions of arbitrary size
      mask Callback mode: bus_expand_callback();
      mask Callback outputWidth: bus_expand_callback();
      mask Callback outputToWorkspace: bus_expand_callback();
  reorder1 : Subsystem  AncestorBlock=casper_library_reorder/reorder  mask(reorder){map=[0 2 1 3], n_bits=64, n_inputs=1, bram_latency=1, map_latency=1, fanout_latency=2, double_buffer=1, bram_map=off, software_controlled=off}
      mask prompts: map "Output Order:"; n_bits "Data width in"; n_inputs "Number of inputs"; bram_latency "BRAM Latency"; map_latency "Map Latency"; fanout_latency "Fanout latency"; double_buffer "Double Buffer"; bram_map "Use BlockRAM for Map"; software_controlled "Use runtime software control"
      mask init:
      | reorder_init(gcb, ...
      |     'map', map, ...
      |     'n_bits', n_bits, ...
      |     'n_inputs', n_inputs, ...
      |     'bram_latency', bram_latency, ...
      |     'map_latency', map_latency, ...
      |     'fanout_latency', fanout_latency, ...
      |     'double_buffer', double_buffer, ...
      |     'bram_map', bram_map, ...
      |     'software_controlled', software_controlled);
      settings: AttributesFormatString=order=2
      mask Help: eval('xlWeb(''http://casper.berkeley.edu/wiki/Reorder'')')
  reorder2 : Subsystem  AncestorBlock=casper_library_reorder/reorder  mask(reorder){map=reshape(permute(reshape([0 : 2*4*2*16*64 - 1], 64, 16, 2, 4, 2), [3 5 1 4 2]), 2*4*2*16*64, 1), n_bits=64, n_inputs=1, bram_latency=3, map_latency=3, fanout_latency=2, double_buffer=0, bram_map=on, software_controlled=off}
      mask prompts: map "Output Order:"; n_bits "Data width in"; n_inputs "Number of inputs"; bram_latency "BRAM Latency"; map_latency "Map Latency"; fanout_latency "Fanout latency"; double_buffer "Double Buffer"; bram_map "Use BlockRAM for Map"; software_controlled "Use runtime software control"
      mask init: same as snap_fengine/chan_reorder/reorder1
      settings: AttributesFormatString=order=45
      mask Help: eval('xlWeb(''http://casper.berkeley.edu/wiki/Reorder'')')
  reorder3 : Subsystem  AncestorBlock=casper_library_reorder/reorder  mask(reorder){map=[0:1023], n_bits=64, n_inputs=1, bram_latency=3, map_latency=3, fanout_latency=2, double_buffer=1, bram_map=on, software_controlled=on}
      mask prompts: map "Output Order:"; n_bits "Data width in"; n_inputs "Number of inputs"; bram_latency "BRAM Latency"; map_latency "Map Latency"; fanout_latency "Fanout latency"; double_buffer "Double Buffer"; bram_map "Use BlockRAM for Map"; software_controlled "Use runtime software control"
      mask init: same as snap_fengine/chan_reorder/reorder1
      settings: AttributesFormatString=order=2
      mask Help: eval('xlWeb(''http://casper.berkeley.edu/wiki/Reorder'')')
  square_transposer : Subsystem  AncestorBlock=casper_library_reorder/square_transposer  mask(square_transposer){n_inputs=2, async=off}
      mask prompts: n_inputs "Number of inputs (2^?):"; async "Aynchronus operation"
      mask init:
      | square_transposer_init(gcb,...
      |     'n_inputs', n_inputs, ...
      |     'async', async);
      settings: AttributesFormatString=n_inputs=2
      mask Help: eval('xlWeb(''http://casper.berkeley.edu/wiki/Square_transposer'')')
  square_transposer1 : Subsystem  AncestorBlock=casper_library_reorder/square_transposer  mask(square_transposer){n_inputs=2, async=off}
      mask prompts: n_inputs "Number of inputs (2^?):"; async "Aynchronus operation"
      mask init:
      | square_transposer_init(gcb,...
      |     'n_inputs', n_inputs, ...
      |     'async', async);
      settings: AttributesFormatString=n_inputs=2
      mask Help: eval('xlWeb(''http://casper.berkeley.edu/wiki/Square_transposer'')')
  square_transposer2 : Subsystem  AncestorBlock=casper_library_reorder/square_transposer  mask(square_transposer){n_inputs=1, async=off}
      mask prompts: n_inputs "Number of inputs (2^?):"; async "Aynchronus operation"
      mask init:
      | square_transposer_init(gcb,...
      |     'n_inputs', n_inputs, ...
      |     'async', async);
      settings: AttributesFormatString=n_inputs=1
      mask Help: eval('xlWeb(''http://casper.berkeley.edu/wiki/Square_transposer'')')
  sync_out : Outport
  dout : Outport  Port=2
  wires:
  Constant/1 -> reorder2/2(en)
  reorder1/3(dout0) -> dout/1
  reorder1/1(sync_out) -> sync_out/1
  bus_expand/2(out3) -> square_transposer/3(in1)
  bus_expand/4(lsb_out1) -> square_transposer/5(in3)
  bus_expand/3(out2) -> square_transposer/4(in2)
  bus_expand/1(msb_out4) -> square_transposer/2(in0)
  square_transposer/1(sync_out) -> square_transposer2/1(sync)
  square_transposer/2(out0) -> bus_create/1(in1)
  square_transposer/3(out1) -> bus_create/2(in2)
  square_transposer/4(out2) -> bus_create/3(in3)
  square_transposer/5(out3) -> bus_create/4(in4)
  bus_expand1/1(msb_out2) -> bus_expand/1(bus_in)
  reorder2/1(sync_out) -> square_transposer1/1(sync), square_transposer/1(sync)
  bus_expand2/2(out3) -> square_transposer1/3(in1)
  bus_expand2/4(lsb_out1) -> square_transposer1/5(in3)
  bus_expand2/3(out2) -> square_transposer1/4(in2)
  bus_expand2/1(msb_out4) -> square_transposer1/2(in0)
  square_transposer1/2(out0) -> bus_create1/1(in1)
  square_transposer1/3(out1) -> bus_create1/2(in2)
  square_transposer1/4(out2) -> bus_create1/3(in3)
  square_transposer1/5(out3) -> bus_create1/4(in4)
  bus_expand1/2(lsb_out1) -> bus_expand2/1(bus_in)
  bus_create/1(bus_out) -> square_transposer2/2(in0)
  bus_create1/1(bus_out) -> square_transposer2/3(in1)
  square_transposer2/1(sync_out) -> reorder1/1(sync)
  square_transposer2/3(out1) -> bus_create2/2(in2)
  square_transposer2/2(out0) -> bus_create2/1(in1)
  reorder2/3(dout0) -> bus_expand1/1(bus_in)
  Constant1/1 -> reorder1/2(en)
  bus_create2/1(bus_out) -> reorder1/3(din0)
  Constant2/1 -> reorder3/2(en)
  sync/1 -> reorder3/1(sync)
  din/1 -> reorder3/3(din0)
  reorder3/2(valid) -> ?
  reorder3/3(dout0) -> reorder2/3(din0)
  reorder3/1(sync_out) -> reorder2/1(sync)

== system snap_fengine/corr ==
  sync : Inport
  din : Inport  Port=2
  0 : Subsystem  mask{nchan_bits=13, npol_bits=3}
      mask prompts: nchan_bits "Number of channels (2^?)"; npol_bits "Number of pols (2^?)"
  wires:
  sync/1 -> 0/1(sync)
  din/1 -> 0/2(din)

== system snap_fengine/delay ==
  sync : Inport
  din : Inport  Port=2
  Delay1 : xbsIndex_r4/Delay  rst=off  infoeditControl=Selection of Reset will increase slice count due to use of real FFs and instead of SRLs  en=off  latency=1  reg_retiming=on  dbl_ovrd=off  block_type=delay
  delayer : Subsystem
  delays : Subsystem  Tag=xps:sw_reg  AncestorBlock=xps_library/software_register  mask(swreg){io_dir=From Processor, io_delay=0, sample_period=1, names=reg, bitwidths=32, bin_pts=0, arith_types=0, sim_port=on, show_format=off}
      mask prompts: io_dir "I/O direction"; io_delay "I/O delay"; sample_period "Sample period"; names "Bitfield names [msb...lsb]"; bitwidths "Bitfield widths"; bin_pts "Bitfield binary pts"; arith_types "Bitfield types, ufix=0, fix=1, bool=2"; sim_port "Provide sim input/output?"; show_format "Print format string?"
      mask help: A 32-bit software-accessible register. Can be divided into bitfields of varying widths and types using the fields in the block mask.
      mask init:
      | swreg_init(gcb)
      settings: AttributesFormatString=1input
      mask TypeOptions io_dir: To Processor | From Processor
      mask Callback io_dir:
      | mask_enables = get_param(gcb, 'MaskEnables');
      | mask_names = get_param(gcb, 'MaskNames');
      | if strcmp(get_param(gcb, 'io_dir'), 'To Processor'),
      |     mask_enables{ismember(mask_names, 'sample_period')} = 'off';
      | else
      |     mask_enables{ismember(mask_names, 'sample_period')} = 'on';
      | end
      | set_param(gcb, 'MaskEnables', mask_enables);
  sync_out : Outport
  dout : Outport  Port=2
  wires:
  delays/1(in_reg) -> delayer/1(delays)
  din/1 -> delayer/2(din)
  delayer/1(dout) -> dout/1
  sync/1 -> Delay1/1
  Delay1/1 -> sync_out/1

== system snap_fengine/eq ==
  note: After quantizing, do the final stage of the FFT descramble.
      | With 4-, rather than 18-bit values, it'll use 25% of the BRAM.
  sync : Inport
  din : Inport  Port=2
  Constant : xbsIndex_r4/Constant  const=1  gui_display_data_type=Boolean  arith_type=Boolean  n_bits=1  bin_pt=0  preci_type=Single  exp_width=8  frac_width=24  explicit_period=on  period=1  equ=P=C  opselect=C  inp2=PCIN>>17  opr=+  inp1=P  carry=CIN  dbl_ovrd=off  block_type=constant
  core : Subsystem  mask{nchan=13-3, nants=8}
      mask prompts: nchan "Number of fft channels (2^?)"; nants "Number of Antennas"
  reorder : Subsystem  AncestorBlock=casper_library_reorder/reorder  mask(reorder){map=[0 8 16 24 32 40 48 56 64 72 80 88 96 104 112 120 128 136 144 152 160 168 176 184 192 200 208 216 224 232 240 248 256 264 272 280 288 296 304 312 320 328 336 344 352 360 368 376 384 392 400 408 416 424 432 440 448 456 464 472 480 488 496 504 512 520 528 536 544 552 560 568 576 584 592 600 608 616 624 632 640 648 656 664 672 680 688 696 704 712 720 728 736 744 752 760 768 776 784 792 800 808 816 824 832 840 848 856 864 872 880 888 896 904 912 920 928 936 944 952 960 968 976 984 992 1000 1008 1016 1 9 17 25 33 41 49 57 65 73 81 89 97 105 113 121 129 137 145 153 161 169 177 185 193 201 209 217 225 233 241 249 257 265 273 281 289 297 305 313 321 329 337 345 353 361 369 377 385 393 401 409 417 425 433 441 449 457 465 473 481 489 497 505 513 521 529 537 545 553 561 569 577 585 593 601 609 617 625 633 641 649 657 665 673 681 689 697 705 713 721 729 737 745 753 761 769 777 785 793 801 809 817 825 833 841 849 857 865 873 881 889 897 905 913 921 929 937 945 953 961 969 977 985 993 1001 1009 1017 2 10 18 26 34 42 50 58 66 74 82 90 98 106 114 122 130 138 146 154 162 170 178 186 194 202 210 218 226 234 242 250 258 266 274 282 290 298 306 314 322 330 338 346 354 362 370 378 386 394 402 410 418 426 434 442 450 458 466 474 482 490 498 506 514 522 530 538 546 554 562 570 578 586 594 602 610 618 626 634 642 650 658 666 674 682 690 698 706 714 722 730 738 746 754 762 770 778 786 794 802 810 818 826 834 842 850 858 866 874 882 890 898 906 914 922 930 938 946 954 962 970 978 986 994 1002 1010 1018 3 11 19 27 35 43 51 59 67 75 83 91 99 107 115 123 131 139 147 155 163 171 179 187 195 203 211 219 227 235 243 251 259 267 275 283 291 299 307 315 323 331 339 347 355 363 371 379 387 395 403 411 419 427 435 443 451 459 467 475 483 491 499 507 515 523 531 539 547 555 563 571 579 587 595 603 611 619 627 635 643 651 659 667 675 683 691 699 707 715 723 731 739 747 755 763 771 779 787 795 803 811 819 827 835 843 851 859 867 875 883 891 899 907 915 923 931 939 947 955 963 971 979 987 995 1003 1011 1019 4 12 20 28 36 44 52 60 68 76 84 92 100 108 116 124 132 140 148 156 164 172 180 188 196 204 212 220 228 236 244 252 260 268 276 284 292 300 308 316 324 332 340 348 356 364 372 380 388 396 404 412 420 428 436 444 452 460 468 476 484 492 500 508 516 524 532 540 548 556 564 572 580 588 596 604 612 620 628 636 644 652 660 668 676 684 692 700 708 716 724 732 740 748 756 764 772 780 788 796 804 812 820 828 836 844 852 860 868 876 884 892 900 908 916 924 932 940 948 956 964 972 980 988 996 1004 1012 1020 5 13 21 29 37 45 53 61 69 77 85 93 101 109 117 125 133 141 149 157 165 173 181 189 197 205 213 221 229 237 245 253 261 269 277 285 293 301 309 317 325 333 341 349 357 365 373 381 389 397 405 413 421 429 437 445 453 461 469 477 485 493 501 509 517 525 533 541 549 557 565 573 581 589 597 605 613 621 629 637 645 653 661 669 677 685 693 701 709 717 725 733 741 749 757 765 773 781 789 797 805 813 821 829 837 845 853 861 869 877 885 893 901 909 917 925 933 941 949 957 965 973 981 989 997 1005 1013 1021 6 14 22 30 38 46 54 62 70 78 86 94 102 110 118 126 134 142 150 158 166 174 182 190 198 206 214 222 230 238 246 254 262 270 278 286 294 302 310 318 326 334 342 350 358 366 374 382 390 398 406 414 422 430 438 446 454 462 470 478 486 494 502 510 518 526 534 542 550 558 566 574 582 590 598 606 614 622 630 638 646 654 662 670 678 686 694 702 710 718 726 734 742 750 758 766 774 782 790 798 806 814 822 830 838 846 854 862 870 878 886 894 902 910 918 926 934 942 950 958 966 974 982 990 998 1006 1014 1022 7 15 23 31 39 47 55 63 71 79 87 95 103 111 119 127 135 143 151 159 167 175 183 191 199 207 215 223 231 239 247 255 263 271 279 287 295 303 311 319 327 335 343 351 359 367 375 383 391 399 407 415 423 431 439 447 455 463 471 479 487 495 503 511 519 527 535 543 551 559 567 575 583 591 599 607 615 623 631 639 647 655 663 671 679 687 695 703 711 719 727 735 743 751 759 767 775 783 791 799 807 815 823 831 839 847 855 863 871 879 887 895 903 911 919 927 935 943 951 959 967 975 983 991 999 1007 1015 1023], n_bits=64, n_inputs=1, bram_latency=3, map_latency=1, fanout_latency=1, double_buffer=0, bram_map=on, software_controlled=off}
      mask prompts: map "Output Order:"; n_bits "Data width in"; n_inputs "Number of inputs"; bram_latency "BRAM Latency"; map_latency "Map Latency"; fanout_latency "Fanout latency"; double_buffer "Double Buffer"; bram_map "Use BlockRAM for Map"; software_controlled "Use runtime software control"
      mask init: same as snap_fengine/chan_reorder/reorder1
      settings: AttributesFormatString=order=10
      mask Help: eval('xlWeb(''http://casper.berkeley.edu/wiki/Reorder'')')
  sync_out : Outport
  dout : Outport  Port=2
  wires:
  din/1 -> core/2(in)
  sync/1 -> core/1(sync)
  Constant/1 -> reorder/2(en)
  core/1(sync_out) -> reorder/1(sync)
  core/2(dout) -> reorder/3(din0)  "data"
  reorder/1(sync_out) -> sync_out/1
  reorder/3(dout0) -> dout/1
